simulink model "VIRTTAC_Model"  (Simulink 7.0)
settings: Solver=ode4  StartTime=VIRTTAC.Sim.StartTime  StopTime=VIRTTAC.Sim.EndTime  FixedStep=VIRTTAC.Sim.SampleTime  RelTol=1e-3
undefined symbols (not defined in the file or in its folder): VIRTTAC
libraries: VIRTTAC_Castor x1
settings Model: Creator=deil_ch  LastModifiedBy=feza_ni
settings DataIOCC: LimitDataPoints=off
settings DebuggingCC: SignalInfNanChecking=error  SolverPrmCheckMsg=none  DiscreteInheritContinuousMsg=error  SingleTaskRateTransMsg=error  TasksWithSamePriorityMsg=error  SigSpecEnsureSampleTimeMsg=error  CheckMatrixSingularityMsg=error  UnconnectedInputMsg=error  UnconnectedOutputMsg=error  UnconnectedLineMsg=error  BusObjectLabelMismatch=error  RootOutportRequireBusObject=error  StrictBusMsg=ErrorOnBusTreatedAsVector

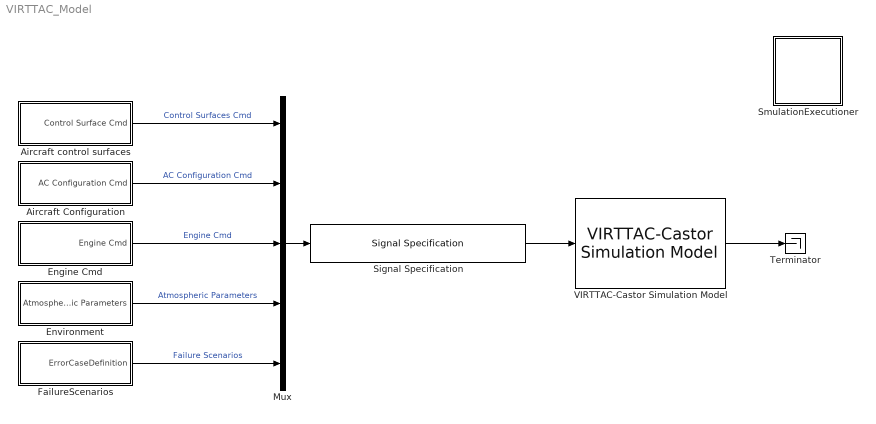
== system VIRTTAC_Model ==
  Aircraft Configuration : Subsystem
  Aircraft control surfaces : Subsystem
  Engine Cmd : Subsystem
  Environment : Subsystem
  FailureScenarios : Subsystem
  Mux : Mux  Inputs=5
  Signal Specification : SignalSpecification  Dimensions=VIRTTAC.Sim.InputPortDim  DataType=double  OutDataType=sfix(16)  OutScaling=2^0
  SmulationExecutioner : Subsystem
  Terminator : Terminator
  VIRTTAC-Castor Simulation Model : VIRTTAC_Castor/VIRTTAC-Castor Simulation Model  SystemSampleTime=-1
  wires:
  Mux/1 -> Signal Specification/1
  Aircraft control surfaces/1(Control Surface Cmd) -> Mux/1  "Control Surfaces Cmd"
  Aircraft Configuration/1(AC Configuration Cmd) -> Mux/2  "AC Configuration Cmd"
  Engine Cmd/1(Engine Cmd) -> Mux/3  "Engine Cmd"
  Environment/1(Atmospheric Parameters) -> Mux/4  "Atmospheric Parameters"
  FailureScenarios/1(ErrorCaseDefinition) -> Mux/5  "Failure Scenarios"
  VIRTTAC-Castor Simulation Model/1 -> Terminator/1
  Signal Specification/1 -> VIRTTAC-Castor Simulation Model/1

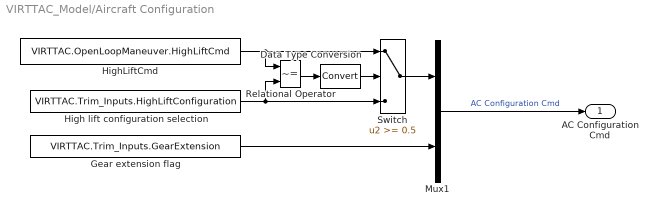
== system VIRTTAC_Model/Aircraft Configuration ==
  Data Type Conversion : DataTypeConversion  OutDataTypeMode=double  OutDataType=sfix(16)  OutScaling=2^0
  Gear extension flag : Constant  Value=VIRTTAC.Trim_Inputs.GearExtension  OutDataType=sfix(16)  OutScaling=2^0
  High lift configuration selection : Constant  Value=VIRTTAC.Trim_Inputs.HighLiftConfiguration  OutDataType=sfix(16)  OutScaling=2^0
  HighLiftCmd : FromWorkspace  VariableName=VIRTTAC.OpenLoopManeuver.HighLiftCmd  SampleTime=0
  Mux1 : Mux  Inputs=2
  Relational Operator : RelationalOperator  Operator=~=  LogicOutDataTypeMode=boolean
  Switch : Switch  Threshold=0.5  OutDataType=sfix(16)  OutScaling=2^0
  AC Configuration Cmd : Outport  PortDimensions=2  DataType=double
  wires:
  Gear extension flag/1 -> Mux1/2
  Mux1/1 -> AC Configuration Cmd/1  "AC Configuration Cmd"
  High lift configuration selection/1 -> Switch/3, Relational Operator/2
  Switch/1 -> Mux1/1
  HighLiftCmd/1 -> Relational Operator/1, Switch/1
  Relational Operator/1 -> Data Type Conversion/1
  Data Type Conversion/1 -> Switch/2

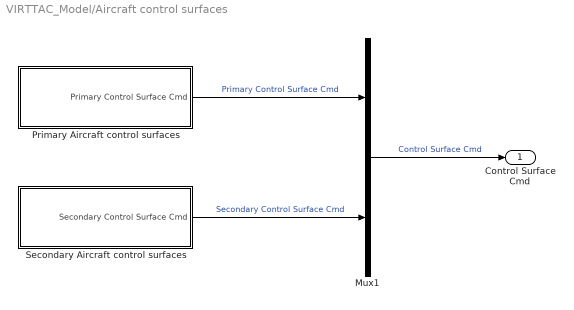
== system VIRTTAC_Model/Aircraft control surfaces ==
  Mux1 : Mux  Inputs=2
  Primary Aircraft control surfaces : Subsystem
  Secondary Aircraft control surfaces : Subsystem
  Control Surface Cmd : Outport  PortDimensions=16  DataType=double
  wires:
  Mux1/1 -> Control Surface Cmd/1  "Control Surface Cmd"
  Primary Aircraft control surfaces/1(Primary Control Surface Cmd) -> Mux1/1  "Primary Control Surface Cmd"
  Secondary Aircraft control surfaces/1(Secondary Control Surface Cmd) -> Mux1/2  "Secondary Control Surface Cmd"

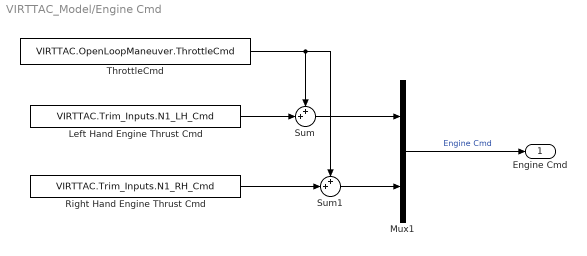
== system VIRTTAC_Model/Engine Cmd ==
  Left Hand Engine Thrust Cmd : Constant  Value=VIRTTAC.Trim_Inputs.N1_LH_Cmd  OutDataType=sfix(16)  OutScaling=2^0
  Mux1 : Mux  Inputs=2
  Right Hand Engine Thrust Cmd : Constant  Value=VIRTTAC.Trim_Inputs.N1_RH_Cmd  OutDataType=sfix(16)  OutScaling=2^0
  Sum : Sum  Inputs=++|  OutDataType=sfix(16)  OutScaling=2^0
  Sum1 : Sum  Inputs=++|  OutDataType=sfix(16)  OutScaling=2^0
  ThrottleCmd : FromWorkspace  VariableName=VIRTTAC.OpenLoopManeuver.ThrottleCmd  SampleTime=0
  Engine Cmd : Outport  PortDimensions=2  DataType=double
  wires:
  Mux1/1 -> Engine Cmd/1  "Engine Cmd"
  Right Hand Engine Thrust Cmd/1 -> Sum1/2
  Left Hand Engine Thrust Cmd/1 -> Sum/2
  Sum/1 -> Mux1/1
  Sum1/1 -> Mux1/2
  ThrottleCmd/1 -> Sum/1, Sum1/1

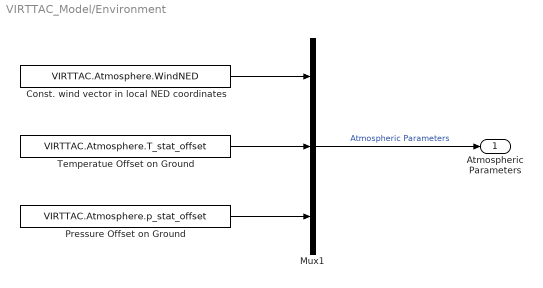
== system VIRTTAC_Model/Environment ==
  Const. wind vector in local NED coordinates : Constant  Value=VIRTTAC.Atmosphere.WindNED  OutDataType=sfix(16)  OutScaling=2^0
  Mux1 : Mux  Inputs=3
  Pressure Offset on Ground : Constant  Value=VIRTTAC.Atmosphere.p_stat_offset  OutDataType=sfix(16)  OutScaling=2^0
  Temperatue Offset on Ground : Constant  Value=VIRTTAC.Atmosphere.T_stat_offset  OutDataType=sfix(16)  OutScaling=2^0
  Atmospheric Parameters : Outport  PortDimensions=5  DataType=double
  wires:
  Mux1/1 -> Atmospheric Parameters/1  "Atmospheric Parameters"
  Pressure Offset on Ground/1 -> Mux1/3
  Temperatue Offset on Ground/1 -> Mux1/2
  Const. wind vector in local NED coordinates/1 -> Mux1/1

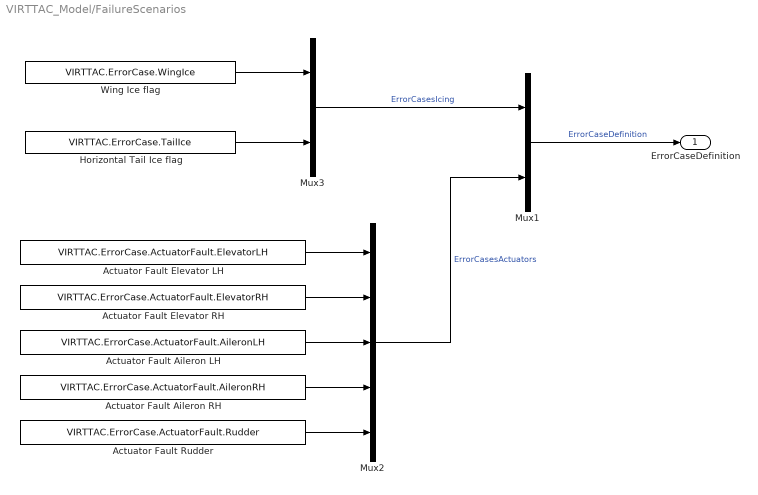
== system VIRTTAC_Model/FailureScenarios ==
  Actuator Fault Aileron LH : Constant  Value=VIRTTAC.ErrorCase.ActuatorFault.AileronLH  OutDataType=sfix(16)  OutScaling=2^0
  Actuator Fault Aileron RH : Constant  Value=VIRTTAC.ErrorCase.ActuatorFault.AileronRH  OutDataType=sfix(16)  OutScaling=2^0
  Actuator Fault Elevator LH : Constant  Value=VIRTTAC.ErrorCase.ActuatorFault.ElevatorLH  OutDataType=sfix(16)  OutScaling=2^0
  Actuator Fault Elevator RH : Constant  Value=VIRTTAC.ErrorCase.ActuatorFault.ElevatorRH  OutDataType=sfix(16)  OutScaling=2^0
  Actuator Fault Rudder : Constant  Value=VIRTTAC.ErrorCase.ActuatorFault.Rudder  OutDataType=sfix(16)  OutScaling=2^0
  Horizontal Tail Ice flag : Constant  Value=VIRTTAC.ErrorCase.TailIce  OutDataType=sfix(16)  OutScaling=2^0
  Mux1 : Mux  Inputs=2
  Mux2 : Mux  Inputs=5
  Mux3 : Mux  Inputs=2
  Wing Ice flag : Constant  Value=VIRTTAC.ErrorCase.WingIce  OutDataType=sfix(16)  OutScaling=2^0
  ErrorCaseDefinition : Outport  PortDimensions=7  DataType=double
  wires:
  Mux1/1 -> ErrorCaseDefinition/1  "ErrorCaseDefinition"
  Actuator Fault Elevator LH/1 -> Mux2/1
  Actuator Fault Elevator RH/1 -> Mux2/2
  Actuator Fault Aileron LH/1 -> Mux2/3
  Actuator Fault Aileron RH/1 -> Mux2/4
  Actuator Fault Rudder/1 -> Mux2/5
  Wing Ice flag/1 -> Mux3/1
  Horizontal Tail Ice flag/1 -> Mux3/2
  Mux3/1 -> Mux1/1  "ErrorCasesIcing"
  Mux2/1 -> Mux1/2  "ErrorCasesActuators"

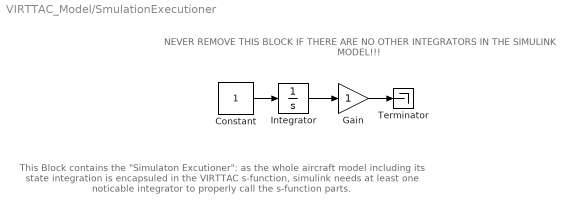
== system VIRTTAC_Model/SmulationExecutioner ==
  note: This Block contains the "Simulaton Excutioner":
      | as the whole aircraft model including its state integration
      | is encapsuled in the VIRTTAC s-function, simulink needs
      | at least one noticable integrator to properly call
      | the s-function parts.
  note: NEVER REMOVE THIS BLOCK IF THERE ARE
      | NO OTHER INTEGRATORS IN THE SIMULINK MODEL!!!
  Constant : Constant  OutDataType=sfix(16)  OutScaling=2^0
  Gain : Gain  ParameterDataType=sfix(16)  ParameterScaling=2^0  OutDataType=sfix(16)  OutScaling=2^0
  Integrator : Integrator
  Terminator : Terminator
  wires:
  Constant/1 -> Integrator/1
  Integrator/1 -> Gain/1
  Gain/1 -> Terminator/1

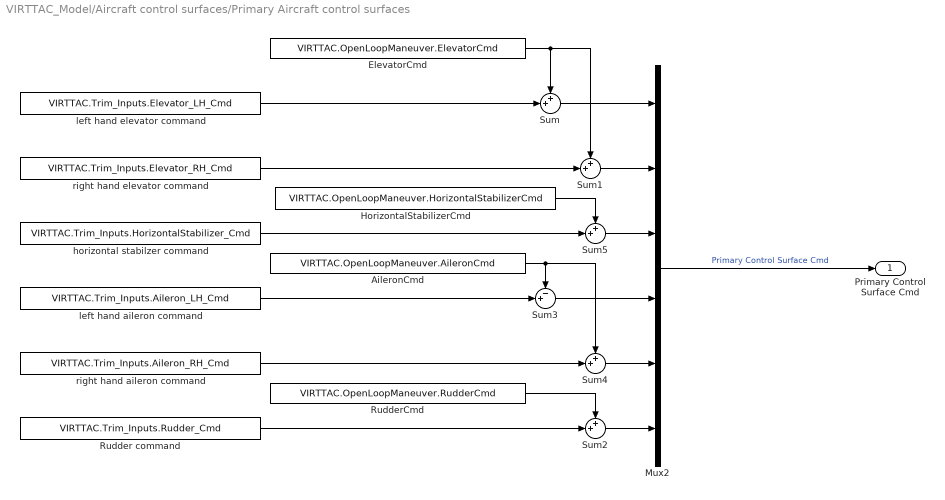
== system VIRTTAC_Model/Aircraft control surfaces/Primary Aircraft control surfaces ==
  AileronCmd : FromWorkspace  VariableName=VIRTTAC.OpenLoopManeuver.AileronCmd  SampleTime=0
  ElevatorCmd : FromWorkspace  VariableName=VIRTTAC.OpenLoopManeuver.ElevatorCmd  SampleTime=0
  HorizontalStabilizerCmd : FromWorkspace  VariableName=VIRTTAC.OpenLoopManeuver.HorizontalStabilizerCmd  SampleTime=0
  Mux2 : Mux  Inputs=6
  Rudder command : Constant  Value=VIRTTAC.Trim_Inputs.Rudder_Cmd  OutDataType=sfix(16)  OutScaling=2^0
  RudderCmd : FromWorkspace  VariableName=VIRTTAC.OpenLoopManeuver.RudderCmd  SampleTime=0
  Sum{,1..2,4..5} (5 alike) : Sum  Inputs=++|  OutDataType=sfix(16)  OutScaling=2^0
  Sum3 : Sum  Inputs=-+|  OutDataType=sfix(16)  OutScaling=2^0
  horizontal stabilzer command : Constant  Value=VIRTTAC.Trim_Inputs.HorizontalStabilizer_Cmd  OutDataType=sfix(16)  OutScaling=2^0
  left hand aileron command : Constant  Value=VIRTTAC.Trim_Inputs.Aileron_LH_Cmd  OutDataType=sfix(16)  OutScaling=2^0
  left hand elevator command : Constant  Value=VIRTTAC.Trim_Inputs.Elevator_LH_Cmd  OutDataType=sfix(16)  OutScaling=2^0
  right hand aileron command : Constant  Value=VIRTTAC.Trim_Inputs.Aileron_RH_Cmd  OutDataType=sfix(16)  OutScaling=2^0
  right hand elevator command : Constant  Value=VIRTTAC.Trim_Inputs.Elevator_RH_Cmd  OutDataType=sfix(16)  OutScaling=2^0
  Primary Control Surface Cmd : Outport  PortDimensions=6  DataType=double
  wires:
  left hand elevator command/1 -> Sum/2
  right hand elevator command/1 -> Sum1/2
  Mux2/1 -> Primary Control Surface Cmd/1  "Primary Control Surface Cmd"
  Rudder command/1 -> Sum2/2
  right hand aileron command/1 -> Sum4/2
  horizontal stabilzer command/1 -> Sum5/2
  ElevatorCmd/1 -> Sum/1, Sum1/1
  Sum/1 -> Mux2/1
  Sum1/1 -> Mux2/2
  Sum2/1 -> Mux2/6
  RudderCmd/1 -> Sum2/1
  Sum4/1 -> Mux2/5
  left hand aileron command/1 -> Sum3/2
  Sum3/1 -> Mux2/4
  AileronCmd/1 -> Sum3/1, Sum4/1
  Sum5/1 -> Mux2/3
  HorizontalStabilizerCmd/1 -> Sum5/1

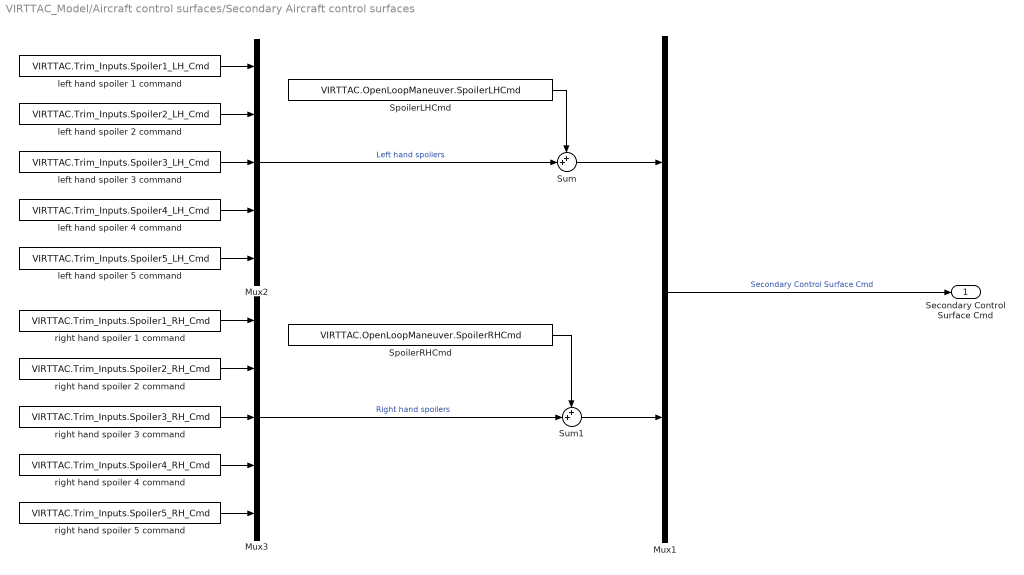
== system VIRTTAC_Model/Aircraft control surfaces/Secondary Aircraft control surfaces ==
  Mux1 : Mux  Inputs=2
  Mux2 : Mux  Inputs=5
  Mux3 : Mux  Inputs=5
  SpoilerLHCmd : FromWorkspace  VariableName=VIRTTAC.OpenLoopManeuver.SpoilerLHCmd  SampleTime=0
  SpoilerRHCmd : FromWorkspace  VariableName=VIRTTAC.OpenLoopManeuver.SpoilerRHCmd  SampleTime=0
  Sum : Sum  Inputs=++|  OutDataType=sfix(16)  OutScaling=2^0
  Sum1 : Sum  Inputs=++|  OutDataType=sfix(16)  OutScaling=2^0
  left hand spoiler 1 command : Constant  Value=VIRTTAC.Trim_Inputs.Spoiler1_LH_Cmd  OutDataType=sfix(16)  OutScaling=2^0
  left hand spoiler 2 command : Constant  Value=VIRTTAC.Trim_Inputs.Spoiler2_LH_Cmd  OutDataType=sfix(16)  OutScaling=2^0
  left hand spoiler 3 command : Constant  Value=VIRTTAC.Trim_Inputs.Spoiler3_LH_Cmd  OutDataType=sfix(16)  OutScaling=2^0
  left hand spoiler 4 command : Constant  Value=VIRTTAC.Trim_Inputs.Spoiler4_LH_Cmd  OutDataType=sfix(16)  OutScaling=2^0
  left hand spoiler 5 command : Constant  Value=VIRTTAC.Trim_Inputs.Spoiler5_LH_Cmd  OutDataType=sfix(16)  OutScaling=2^0
  right hand spoiler 1 command : Constant  Value=VIRTTAC.Trim_Inputs.Spoiler1_RH_Cmd  OutDataType=sfix(16)  OutScaling=2^0
  right hand spoiler 2 command : Constant  Value=VIRTTAC.Trim_Inputs.Spoiler2_RH_Cmd  OutDataType=sfix(16)  OutScaling=2^0
  right hand spoiler 3 command : Constant  Value=VIRTTAC.Trim_Inputs.Spoiler3_RH_Cmd  OutDataType=sfix(16)  OutScaling=2^0
  right hand spoiler 4 command : Constant  Value=VIRTTAC.Trim_Inputs.Spoiler4_RH_Cmd  OutDataType=sfix(16)  OutScaling=2^0
  right hand spoiler 5 command : Constant  Value=VIRTTAC.Trim_Inputs.Spoiler5_RH_Cmd  OutDataType=sfix(16)  OutScaling=2^0
  Secondary Control Surface Cmd : Outport  PortDimensions=10  DataType=double
  wires:
  Mux1/1 -> Secondary Control Surface Cmd/1  "Secondary Control Surface Cmd"
  left hand spoiler 5 command/1 -> Mux2/5
  left hand spoiler 4 command/1 -> Mux2/4
  left hand spoiler 3 command/1 -> Mux2/3
  left hand spoiler 2 command/1 -> Mux2/2
  left hand spoiler 1 command/1 -> Mux2/1
  Mux2/1 -> Sum/2  "Left hand spoilers"
  Mux3/1 -> Sum1/2  "Right hand spoilers"
  right hand spoiler 1 command/1 -> Mux3/1
  right hand spoiler 2 command/1 -> Mux3/2
  right hand spoiler 3 command/1 -> Mux3/3
  right hand spoiler 4 command/1 -> Mux3/4
  right hand spoiler 5 command/1 -> Mux3/5
  Sum/1 -> Mux1/1
  SpoilerLHCmd/1 -> Sum/1
  SpoilerRHCmd/1 -> Sum1/1
  Sum1/1 -> Mux1/2
